simulink model "Simulink_recibir_datos"  (R2025b)
settings: Solver=VariableStepAuto  StartTime=0.0  StopTime=Inf  RelTol=1e-3
libraries: instrumentseriallib x2
settings Model: Creator=Claudio  LastModifiedBy=bianc
settings DebuggingCC: UnconnectedInputMsg=warning  UnconnectedOutputMsg=warning  UnconnectedLineMsg=warning
settings ModelReferenceCC: EnableRefExpFcnMdlSchedulingChecks=on
settings RTWCC: GPUComputeCapability=3.5  DLArmComputeVersion=19.05

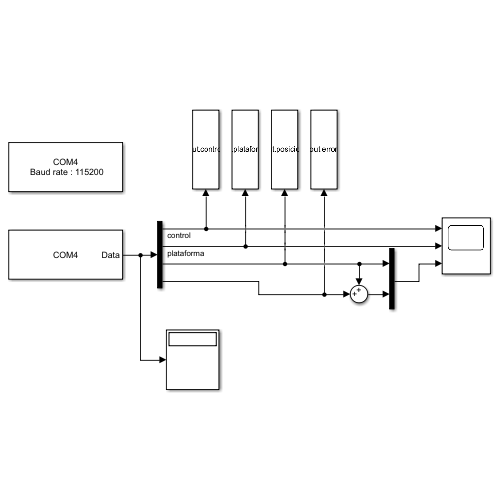
[thumbnail: Simulink's stored preview of the top-level diagram]
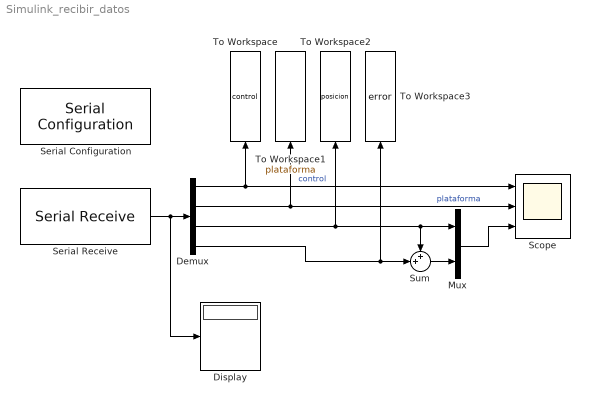
== system Simulink_recibir_datos ==
  Demux : Demux
  Display : Display
  Mux : Mux  Inputs=2
  Scope : Scope  NumInputPorts=3
      settings: TimeSpan=60  ActiveDisplayYMinimum=-3.7499999999999991  ActiveDisplayYMaximum=33.75
  Serial Configuration : instrumentseriallib/Serial Configuration  Priority=-200000  PortSel=COM4  Port=COM4  ComPort=COM4  BaudRate=115200  DataBits=8  Parity=none  StopBits=1  ByteOrder=big-endian  FlowControl=none  Timeout=10  SimulateUsing=Interpreted execution  BlockInModel=on  aMode=1
  Serial Receive : instrumentseriallib/Serial Receive  Priority=1  PortSel=COM4  Port=COM4  ComPort=COM4  DataType=single  SaveDataType=uint8  ToggleHeader=on  Header="[ 97   98   99  100 ]"  ToggleDataSize=on  DataSize=[4 1]  ToggleTerminator=off  Terminator=<none>  CustomTerminator=[]  InputFormat=Column major  EnableBlockingMode=on  ActionDataUnavailable=Output last received value  ActionWhenDataUnavailable=Output last received value  CustomValue=0  SampleTime=0.02  SimulateUsing=Interpreted execution  BlockInModel=on  aMode=1  LibraryInUse=instrumentlib
  Sum : Sum  Inputs=++|
  To Workspace : ToWorkspace  VariableName=control  SampleTime=-1
      settings: Save2DSignal=2-D array (concatenate along first dimension)
  To Workspace1 : ToWorkspace  VariableName=plataforma  SampleTime=-1
      settings: Save2DSignal=2-D array (concatenate along first dimension)
  To Workspace2 : ToWorkspace  VariableName=posicion  SampleTime=-1
      settings: Save2DSignal=2-D array (concatenate along first dimension)
  To Workspace3 : ToWorkspace  VariableName=error  SampleTime=-1
      settings: Save2DSignal=2-D array (concatenate along first dimension)
  wires:
  Serial Receive/1 -> Display/1, Demux/1
  Mux/1 -> Scope/3
  Demux/2 -> To Workspace1/1, Scope/2  "plataforma"
  Demux/1 -> To Workspace/1, Scope/1  "control"
  Demux/3 -> To Workspace2/1, Mux/1, Sum/1
  Sum/1 -> Mux/2
  Demux/4 -> To Workspace3/1, Sum/2
